simulink model "demodApproach3"  (R2019b)
settings: Solver=VariableStepAuto  StartTime=0.0  StopTime=0.005  FixedStep=1/2400  MaxStep=.01/2400  RelTol=1e-3
undefined symbols (not defined in the file): DiscIntNeverNeededParam
settings Model: Creator=Pranay  LastModifiedBy=Pranay
settings DebuggingCC: IgnoredZcDiagnostic=none

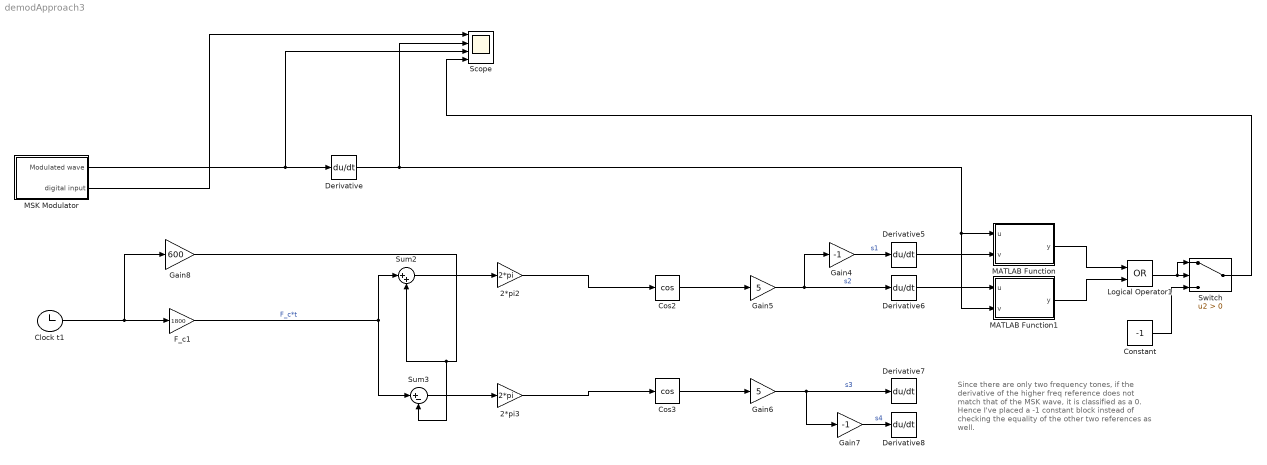
== system demodApproach3 ==
  note: Since there are only two frequency tones, if the derivative of the higher freq reference does not match that of the MSK wave, it is classified as a 0. Hence I've placed a -1 constant block instead of checking the equality of the other two references as well.
  2*pi2 : Gain  Gain=2*pi
  2*pi3 : Gain  Gain=2*pi
  Clock t1 : Clock
  Constant : Constant  Value=-1
  Cos2 : Trigonometry  Operator=cos
  Cos3 : Trigonometry  Operator=cos
  Derivative{,5..8} (5 alike) : Derivative
  F_c1 : Gain  Gain=1800
  Gain4 : Gain  Gain=-1
  Gain5 : Gain  Gain=5
  Gain6 : Gain  Gain=5
  Gain7 : Gain  Gain=-1
  Gain8 : Gain  Gain=600
  Logical Operator1 : Logic  Operator=OR  AllPortsSameDT=off  OutDataTypeStr=boolean
  MATLAB Function : MATLAB Function  TreatAsAtomicUnit=on
  MATLAB Function1 : MATLAB Function  TreatAsAtomicUnit=on
  MSK Modulator : Subsystem
  Scope : Scope  NumInputPorts=4
  Sum2 : Sum  Inputs=|++
  Sum3 : Sum  Inputs=|+-
  Switch : Switch  Criteria=u2 > Threshold  ZeroCross=off
  wires:
  MSK Modulator/1(Modulated wave) -> Scope/3, Derivative/1
  Gain8/1 -> Sum3/2, Sum2/2
  Cos3/1 -> Gain6/1
  Derivative5/1 -> MATLAB Function/2(v)
  Sum3/1 -> 2*pi3/1
  Sum2/1 -> 2*pi2/1
  Gain5/1 -> Derivative6/1, Gain4/1  "s2"
  2*pi2/1 -> Cos2/1
  Gain4/1 -> Derivative5/1  "s1"
  MATLAB Function/1(y) -> Logical Operator1/1
  Gain7/1 -> Derivative8/1  "s4"
  2*pi3/1 -> Cos3/1
  Cos2/1 -> Gain5/1
  F_c1/1 -> Sum3/1, Sum2/1  "F_c*t"
  Clock t1/1 -> Gain8/1, F_c1/1
  Gain6/1 -> Derivative7/1, Gain7/1  "s3"
  Derivative6/1 -> MATLAB Function1/1(u)
  MATLAB Function1/1(y) -> Logical Operator1/2
  Constant/1 -> Switch/3
  Logical Operator1/1 -> Switch/1, Switch/2
  Derivative/1 -> Scope/2, MATLAB Function1/2(v), MATLAB Function/1(u)
  Switch/1 -> Scope/4
  MSK Modulator/2(digital input) -> Scope/1

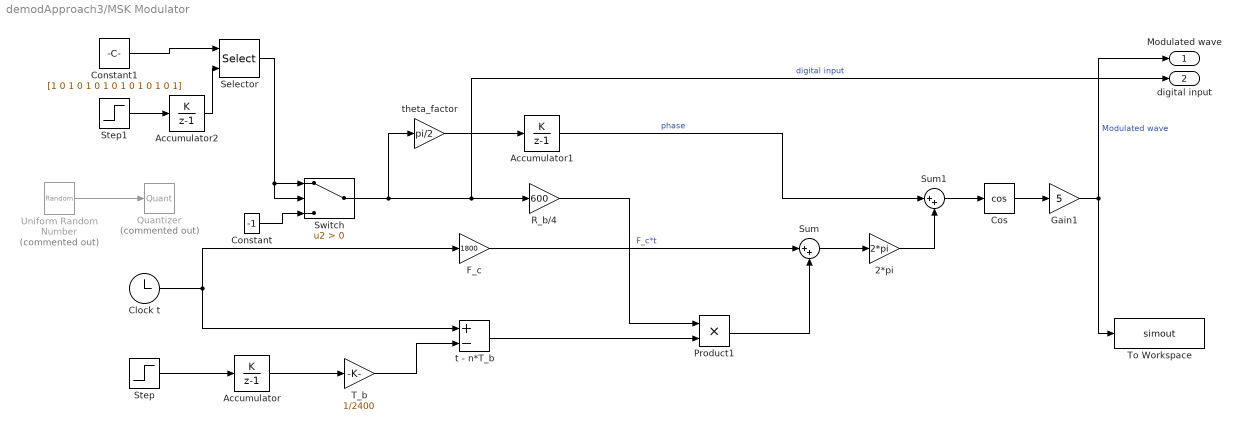
== system demodApproach3/MSK Modulator ==
  2*pi : Gain  Gain=2*pi
  Accumulator : DiscreteIntegrator  IntegratorMethod=Accumulation: Forward Euler  SampleTime=-1  ICPrevOutput=DiscIntNeverNeededParam  ICPrevScaledInput=DiscIntNeverNeededParam
  Accumulator1 : DiscreteIntegrator  IntegratorMethod=Accumulation: Forward Euler  gainval=1  SampleTime=-1  ICPrevOutput=DiscIntNeverNeededParam  ICPrevScaledInput=DiscIntNeverNeededParam
  Accumulator2 : DiscreteIntegrator  IntegratorMethod=Accumulation: Forward Euler  gainval=1  SampleTime=-1  LimitOutput=on  UpperSaturationLimit=14  ICPrevOutput=DiscIntNeverNeededParam  ICPrevScaledInput=DiscIntNeverNeededParam
  Clock t : Clock
  Constant : Constant  Value=-1
  Constant1 : Constant  Value=[1 0 1 0 1 0 1 0 1 0 1 0 1 0 1]
  Cos : Trigonometry  Operator=cos
  F_c : Gain  Gain=1800
  Gain1 : Gain  Gain=5
  Product1 : Product
  Quantizer : Quantizer  Commented=on  QuantizationInterval=1
  R_b/4 : Gain  Gain=600
  Selector : Selector  IndexMode=Zero-based  InputPortWidth=15  IndexOptions=Index vector (port)  Indices=[1 3]  OutputSizes=1
  Step : Step  Time=0  SampleTime=0
  Step1 : Step  Time=0  SampleTime=1/2400
  Sum : Sum  Inputs=|++
  Sum1 : Sum  Inputs=|++
  Switch : Switch  Criteria=u2 > Threshold
  T_b : Gain  Gain=1/2400
  To Workspace : ToWorkspace  VariableName=simout  SampleTime=-1
  Uniform Random Number : UniformRandomNumber  Commented=on  Minimum=0  SampleTime=1/2400
  t - n*T_b : Sum  Inputs=+-
  theta_factor : Gain  Gain=pi/2
  Modulated wave : Outport
  digital input : Outport  Port=2
  wires:
  2*pi/1 -> Sum1/2
  theta_factor/1 -> Accumulator1/1
  Cos/1 -> Gain1/1
  Step/1 -> Accumulator/1
  T_b/1 -> t - n*T_b/2
  Accumulator/1 -> T_b/1
  Constant/1 -> Switch/3
  Sum/1 -> 2*pi/1
  Switch/1 -> theta_factor/1, digital input/1, R_b/4/1  "digital input"
  Clock t/1 -> t - n*T_b/1, F_c/1
  Gain1/1 -> Modulated wave/1, To Workspace/1  "Modulated wave"
  Uniform Random Number/1 -> Quantizer/1
  F_c/1 -> Sum/1  "F_c*t"
  Accumulator1/1 -> Sum1/1  "phase"
  t - n*T_b/1 -> Product1/2
  Product1/1 -> Sum/2
  Sum1/1 -> Cos/1
  R_b/4/1 -> Product1/1
  Constant1/1 -> Selector/1
  Step1/1 -> Accumulator2/1
  Accumulator2/1 -> Selector/2
  Selector/1 -> Switch/1, Switch/2

== matlab function demodApproach3/MATLAB Function1 ==
  data: u input; y output; v input
function y = fcn(u, v)
    diff = abs(u - v);
    if (diff < 0.01)
        t = 1;
    else
        t = 0;
    end
y = t;

== matlab function demodApproach3/MATLAB Function ==
  data: u input; y output; v input
function y = fcn(u, v)
    diff = abs(u - v);
    if (diff < 0.01)
        t = 1;
    else
        t = 0;
    end
y = t;
